simulink model "pos_step_sl"  (R2015a)
settings: Solver=ode3  StartTime=0.0  StopTime=10.0  FixedStep=ts  RelTol=1e-3
values from neighbouring files (symbols this model uses):
  Kp_id = 0.12    [pos_step.m]
  r = 60    [pos_step.m]    (also in sim_init.m; sim_param.mat)
libraries: arduinolib x3
settings Model: SimulationMode=external  ExtModeTrigDuration=2  Creator=shohei  LastModifiedBy=shohei
settings OptimizationCC: OptimizeModelRefInitCode=on  LifeSpan=1
settings DebuggingCC: UnderspecifiedInitializationDetection=Classic  MergeDetectMultiDrivingBlocksExec=none
settings HardwareCC: ProdBitPerInt=16  ProdBitPerPointer=8  ProdIntDivRoundTo=Zero  ProdEndianess=LittleEndian  ProdWordSize=8  ProdHWDeviceType=Atmel->AVR
settings RTWCC: SystemTargetFile=realtime.tlc  GenerateMakefile=off  TemplateMakefile=realtime.tmf  Description=Run on Target Hardware  RTWVerbose=off
settings ERTTargetCC: CombineOutputUpdateFcns=off  ExtModeTransport=3  ExtModeMexFile=ext_serial_win32_comm_rtt  ExtModeMexArgs=0 1 9600  ERTSrcFileBannerTemplate=realtime_code_template.cgt  ERTHdrFileBannerTemplate=realtime_code_template.cgt  ERTDataSrcFileTemplate=realtime_code_template.cgt  ERTDataHdrFileTemplate=realtime_code_template.cgt  ERTCustomFileTemplate=realtime_file_process.tlc

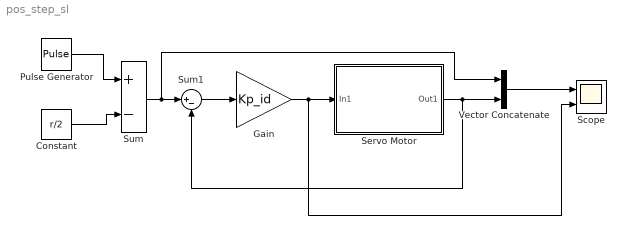
== system pos_step_sl ==
  Constant : Constant  Value=r/2
  Gain : Gain  Gain=Kp_id
  Pulse Generator : DiscretePulseGenerator  PulseType=Time based  Period=10  PulseWidth=50
  Scope : Scope  NumInputPorts=2
      settings: YMin=-30~-3.65  YMax=5~-3.25
  "Servo Motor " : Subsystem
  Sum : Sum  Inputs=+-
  Sum1 : Sum  Inputs=|+-
  Vector Concatenate : Concatenate
  wires:
  Pulse Generator/1 -> Sum/1
  Constant/1 -> Sum/2
  Sum/1 -> Vector Concatenate/1, Sum1/1
  Sum1/1 -> Gain/1
  Gain/1 -> Scope/2, "Servo Motor "/1(In1)
  "Servo Motor "/1(Out1) -> Sum1/2, Vector Concatenate/2
  Vector Concatenate/1 -> Scope/1

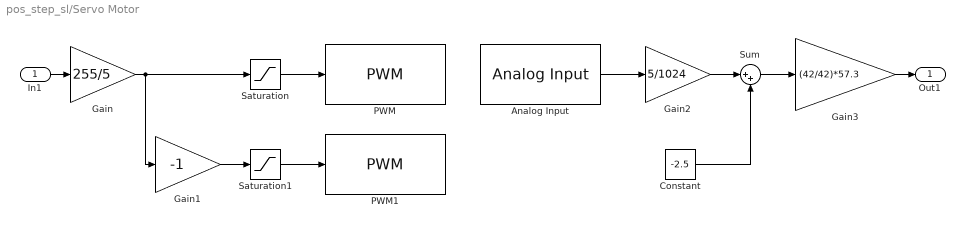
== system pos_step_sl/Servo Motor  ==
  In1 : Inport
  Analog Input : arduinolib/Analog Input  pinNumber=0  sampleTime=ts  blockPlatform=arduino
  Constant : Constant  Value=-2.5
  Gain : Gain  Gain=255/5
  Gain1 : Gain  Gain=-1
  Gain2 : Gain  Gain=5/1024
  Gain3 : Gain  Gain=(42/42)*57.3
  PWM : arduinolib/PWM  pinNumber=3  blockPlatform=arduino
  PWM1 : arduinolib/PWM  pinNumber=5  blockPlatform=arduino
  Saturation : Saturate  UpperLimit=255  LowerLimit=0
  Saturation1 : Saturate  UpperLimit=255  LowerLimit=0
  Sum : Sum  Inputs=|++
  Out1 : Outport
  wires:
  Gain1/1 -> Saturation1/1
  Gain2/1 -> Sum/1
  Sum/1 -> Gain3/1
  Saturation1/1 -> PWM1/1
  Saturation/1 -> PWM/1
  Gain3/1 -> Out1/1
  In1/1 -> Gain/1
  Constant/1 -> Sum/2
  Analog Input/1 -> Gain2/1
  Gain/1 -> Gain1/1, Saturation/1
